simulink model "Airframe"  (R2023b)
settings: Solver=VariableStepAuto  StartTime=0.0  StopTime=10.0  RelTol=1e-3
libraries: cstblocks x2
settings Model: Creator=haita  LastModifiedBy=Albertlakers
settings RTWCC: GPUComputeCapability=5.0

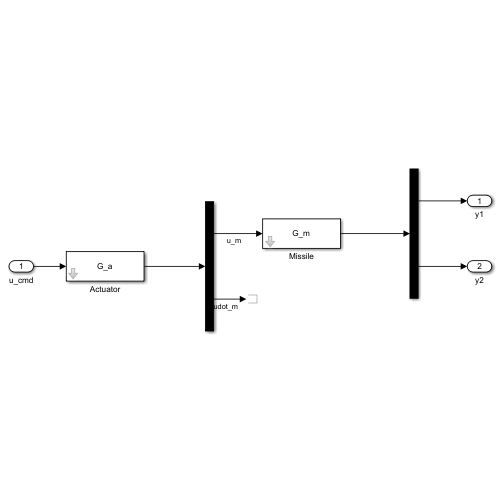
[thumbnail: Simulink's stored preview of the top-level diagram]
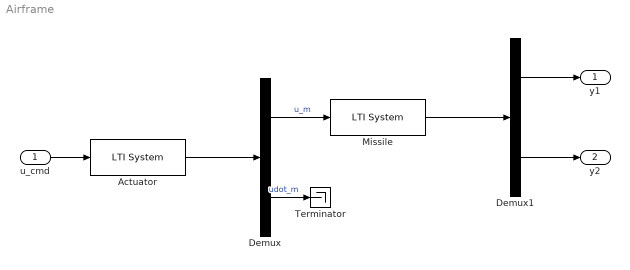
== system Airframe ==
  u_cmd : Inport
  Actuator : cstblocks/LTI System  sys=G_a  IC=[]  PadeOrder=0
  Demux : Demux  Outputs=2
  Demux1 : Demux  Outputs=2
  Missile : cstblocks/LTI System  sys=G_m  IC=[]  PadeOrder=0
  Terminator : Terminator
  y1 : Outport
  y2 : Outport  Port=2
  wires:
  Actuator/1 -> Demux/1
  Demux1/2 -> y2/1
  Demux1/1 -> y1/1
  Demux/1 -> Missile/1  "u_m"
  Missile/1 -> Demux1/1
  u_cmd/1 -> Actuator/1
  Demux/2 -> Terminator/1  "udot_m"
